simulink model "LogicalAccumulatorModel"  (R2020a)
settings: Solver=FixedStepDiscrete  StartTime=0.0  StopTime=400  FixedStep=0.001  RelTol=1e-3
libraries: AccCellGroup x90
settings Model: Creator=sean  LastModifiedBy=sean
settings OptimizationCC: DefaultParameterBehavior=Inlined  UseDivisionForNetSlopeComputation=on  GainParamInheritBuiltInType=on  UseFloatMulNetSlope=on  InlineInvariantSignals=on  PassReuseOutputArgsAs=Individual arguments  ZeroExternalMemoryAtStartup=off  ZeroInternalMemoryAtStartup=off  NoFixptDivByZeroProtection=on  EfficientFloat2IntCast=on  LifeSpan=1  OptimizeBlockOrder=speed  DifferentSizesBufferReuse=on  EfficientTunableParamExpr=on
settings DebuggingCC: ParameterTunabilityLossMsg=error
settings HardwareCC: ProdBitPerLong=64  ProdLongLongMode=on  ProdHWDeviceType=Intel->x86-64 (Linux 64)
settings SFSimCC: MATLABDynamicMemAlloc=off
settings RTWCC: SystemTargetFile=ert.tlc  GenCodeOnly=on  TemplateMakefile=ert_default_tmf
settings CodeAppCC: ForceParamTrailComments=on  IgnoreCustomStorageClasses=off  OperatorAnnotations=on  SimulinkDataObjDesc=on  SFDataObjDesc=on  CustomSymbolStrGlobalVar=rt$N$M  CustomSymbolStrType=$N$M  CustomSymbolStrFcn=$N$M$F  CustomSymbolStrMacro=$N$M  InsertBlockDesc=on
settings ERTTargetCC: TargetLangStandard=C99 (ISO)  GenerateSampleERTMain=on  IncludeMdlTerminateFcn=off  CombineSignalStateStructs=on  SuppressErrorStatus=on  SupportAbsoluteTime=off  SupportComplex=off  InlinedParameterPlacement=NonHierarchical  ERTCustomFileTemplate=example_file_process.tlc  ERTFilePackagingFormat=CompactWithDataFile

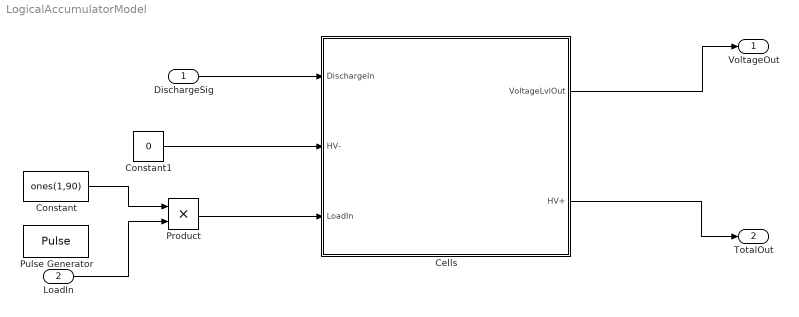
== system LogicalAccumulatorModel ==
  DischargeSig : Inport
  LoadIn : Inport  Port=2
  Cells : Subsystem
  Constant : Constant  Value=ones(1,90)
  Constant1 : Constant  Value=0
  Product : Product
  Pulse Generator : DiscretePulseGenerator  PulseType=Time based  Amplitude=60  Period=300  PulseWidth=99  PhaseDelay=5
  VoltageOut : Outport
  TotalOut : Outport  Port=2
  wires:
  Cells/2(HV+) -> TotalOut/1
  Cells/1(VoltageLvlOut) -> VoltageOut/1
  Constant1/1 -> Cells/2(HV-)
  DischargeSig/1 -> Cells/1(DischargeIn)
  Constant/1 -> Product/1
  Product/1 -> Cells/3(LoadIn)
  LoadIn/1 -> Product/2

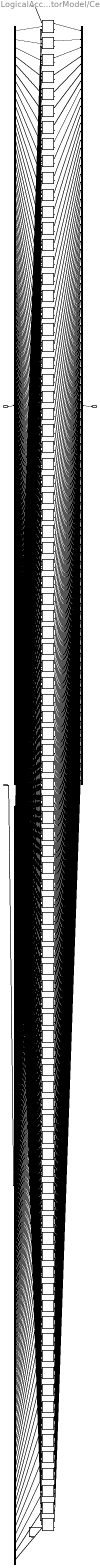
== system LogicalAccumulatorModel/Cells ==
  DischargeIn : Inport
  HV- : Inport  Port=2
  LoadIn : Inport  Port=3
  Cell1 : AccCellGroup/CellGroup  InitialSOCDefficit=0.6400  InternalResistance=0.0018
      settings: SourceProductName=Cell Library
  Cell10 : AccCellGroup/CellGroup  InitialSOCDefficit=0.6500  InternalResistance=0.0018
      settings: SourceProductName=Cell Library
  Cell11 : AccCellGroup/CellGroup  InitialSOCDefficit=0.6100  InternalResistance=0.0018
      settings: SourceProductName=Cell Library
  Cell12 : AccCellGroup/CellGroup  InitialSOCDefficit=0.3900  InternalResistance=0.0018
      settings: SourceProductName=Cell Library
  Cell13 : AccCellGroup/CellGroup  InitialSOCDefficit=0.1400  InternalResistance=0.0018
      settings: SourceProductName=Cell Library
  Cell14 : AccCellGroup/CellGroup  InitialSOCDefficit=0.0200  InternalResistance=0.0018
      settings: SourceProductName=Cell Library
  Cell15 : AccCellGroup/CellGroup  InitialSOCDefficit=0.4200  InternalResistance=0.0018
      settings: SourceProductName=Cell Library
  Cell16 : AccCellGroup/CellGroup  InitialSOCDefficit=0.1800  InternalResistance=0.0018
      settings: SourceProductName=Cell Library
  Cell17 : AccCellGroup/CellGroup  InitialSOCDefficit=0.7300  InternalResistance=0.0018
      settings: SourceProductName=Cell Library
  Cell18 : AccCellGroup/CellGroup  InitialSOCDefficit=0.3700  InternalResistance=0.0018
      settings: SourceProductName=Cell Library
  Cell19 : AccCellGroup/CellGroup  InitialSOCDefficit=0.8400  InternalResistance=0.0018
      settings: SourceProductName=Cell Library
  Cell2 : AccCellGroup/CellGroup  InitialSOCDefficit=0.9600  InternalResistance=0.0018
      settings: SourceProductName=Cell Library
  Cell20 : AccCellGroup/CellGroup  InitialSOCDefficit=0.7400  InternalResistance=0.0018
      settings: SourceProductName=Cell Library
  Cell21 : AccCellGroup/CellGroup  InitialSOCDefficit=0.5700  InternalResistance=0.0018
      settings: SourceProductName=Cell Library
  Cell22 : AccCellGroup/CellGroup  InitialSOCDefficit=0.1700  InternalResistance=0.0018
      settings: SourceProductName=Cell Library
  Cell23 : AccCellGroup/CellGroup  InitialSOCDefficit=0.9600  InternalResistance=0.0018
      settings: SourceProductName=Cell Library
  Cell24 : AccCellGroup/CellGroup  InitialSOCDefficit=0.2600  InternalResistance=0.0018
      settings: SourceProductName=Cell Library
  Cell25 : AccCellGroup/CellGroup  InitialSOCDefficit=0.9300  InternalResistance=0.0018
      settings: SourceProductName=Cell Library
  Cell26 : AccCellGroup/CellGroup  InitialSOCDefficit=0.2200  InternalResistance=0.0018
      settings: SourceProductName=Cell Library
  Cell27 : AccCellGroup/CellGroup  InitialSOCDefficit=0.3700  InternalResistance=0.0018
      settings: SourceProductName=Cell Library
  Cell28 : AccCellGroup/CellGroup  InitialSOCDefficit=0.0800  InternalResistance=0.0018
      settings: SourceProductName=Cell Library
  Cell29 : AccCellGroup/CellGroup  InitialSOCDefficit=0.6400  InternalResistance=0.0018
      settings: SourceProductName=Cell Library
  Cell3 : AccCellGroup/CellGroup  InitialSOCDefficit=0.4400  InternalResistance=0.0018
      settings: SourceProductName=Cell Library
  Cell30 : AccCellGroup/CellGroup  InitialSOCDefficit=0.1800  InternalResistance=0.0018
      settings: SourceProductName=Cell Library
  Cell31 : AccCellGroup/CellGroup  InitialSOCDefficit=0.0400  InternalResistance=0.0018
      settings: SourceProductName=Cell Library
  Cell32 : AccCellGroup/CellGroup  InitialSOCDefficit=0.7300  InternalResistance=0.0018
      settings: SourceProductName=Cell Library
  Cell33 : AccCellGroup/CellGroup  InitialSOCDefficit=0.3500  InternalResistance=0.0018
      settings: SourceProductName=Cell Library
  Cell34 : AccCellGroup/CellGroup  InitialSOCDefficit=0.6600  InternalResistance=0.0018
      settings: SourceProductName=Cell Library
  Cell35 : AccCellGroup/CellGroup  InitialSOCDefficit=0.3800  InternalResistance=0.0018
      settings: SourceProductName=Cell Library
  Cell36 : AccCellGroup/CellGroup  InitialSOCDefficit=0.6300  InternalResistance=0.0018
      settings: SourceProductName=Cell Library
  Cell37 : AccCellGroup/CellGroup  InitialSOCDefficit=0.0200  InternalResistance=0.0018
      settings: SourceProductName=Cell Library
  Cell38 : AccCellGroup/CellGroup  InitialSOCDefficit=0.9100  InternalResistance=0.0018
      settings: SourceProductName=Cell Library
  Cell39 : AccCellGroup/CellGroup  InitialSOCDefficit=0.8000  InternalResistance=0.0018
      settings: SourceProductName=Cell Library
  Cell4 : AccCellGroup/CellGroup  InitialSOCDefficit=0.0600  InternalResistance=0.0018
      settings: SourceProductName=Cell Library
  Cell40 : AccCellGroup/CellGroup  InitialSOCDefficit=0.7500  InternalResistance=0.0018
      settings: SourceProductName=Cell Library
  Cell41 : AccCellGroup/CellGroup  InitialSOCDefficit=0.8200  InternalResistance=0.0018
      settings: SourceProductName=Cell Library
  Cell42 : AccCellGroup/CellGroup  InitialSOCDefficit=0.3800  InternalResistance=0.0018
      settings: SourceProductName=Cell Library
  Cell43 : AccCellGroup/CellGroup  InitialSOCDefficit=0.6200  InternalResistance=0.0018
      settings: SourceProductName=Cell Library
  Cell44 : AccCellGroup/CellGroup  InitialSOCDefficit=0.5800  InternalResistance=0.0018
      settings: SourceProductName=Cell Library
  Cell45 : AccCellGroup/CellGroup  InitialSOCDefficit=0.5300  InternalResistance=0.0018
      settings: SourceProductName=Cell Library
  Cell46 : AccCellGroup/CellGroup  InitialSOCDefficit=0.2700  InternalResistance=0.0018
      settings: SourceProductName=Cell Library
  Cell47 : AccCellGroup/CellGroup  InitialSOCDefficit=0.2500  InternalResistance=0.0018
      settings: SourceProductName=Cell Library
  Cell48 : AccCellGroup/CellGroup  InitialSOCDefficit=0.4500  InternalResistance=0.0018
      settings: SourceProductName=Cell Library
  Cell49 : AccCellGroup/CellGroup  InitialSOCDefficit=0.2200  InternalResistance=0.0018
      settings: SourceProductName=Cell Library
  Cell5 : AccCellGroup/CellGroup  InitialSOCDefficit=0.8700  InternalResistance=0.0018
      settings: SourceProductName=Cell Library
  Cell50 : AccCellGroup/CellGroup  InitialSOCDefficit=0.8100  InternalResistance=0.0018
      settings: SourceProductName=Cell Library
  Cell{51,56,75,78} (4 alike) : AccCellGroup/CellGroup  InitialSOCDefficit=0.9900  InternalResistance=0.0018
      settings: SourceProductName=Cell Library
  Cell52 : AccCellGroup/CellGroup  InitialSOCDefficit=0.0300  InternalResistance=0.0018
      settings: SourceProductName=Cell Library
  Cell53 : AccCellGroup/CellGroup  InitialSOCDefficit=0.5400  InternalResistance=0.0018
      settings: SourceProductName=Cell Library
  Cell54 : AccCellGroup/CellGroup  InitialSOCDefficit=0.0800  InternalResistance=0.0018
      settings: SourceProductName=Cell Library
  Cell55 : AccCellGroup/CellGroup  InitialSOCDefficit=0.8100  InternalResistance=0.0018
      settings: SourceProductName=Cell Library
  Cell57 : AccCellGroup/CellGroup  InitialSOCDefficit=0.0600  InternalResistance=0.0018
      settings: SourceProductName=Cell Library
  Cell58 : AccCellGroup/CellGroup  InitialSOCDefficit=0.9400  InternalResistance=0.0018
      settings: SourceProductName=Cell Library
  Cell59 : AccCellGroup/CellGroup  InitialSOCDefficit=0.0100  InternalResistance=0.0018
      settings: SourceProductName=Cell Library
  Cell6 : AccCellGroup/CellGroup  InitialSOCDefficit=0.6300  InternalResistance=0.0018
      settings: SourceProductName=Cell Library
  Cell60 : AccCellGroup/CellGroup  InitialSOCDefficit=0.6900  InternalResistance=0.0018
      settings: SourceProductName=Cell Library
  Cell61 : AccCellGroup/CellGroup  InitialSOCDefficit=0.7900  InternalResistance=0.0018
      settings: SourceProductName=Cell Library
  Cell62 : AccCellGroup/CellGroup  InitialSOCDefficit=0.5300  InternalResistance=0.0018
      settings: SourceProductName=Cell Library
  Cell63 : AccCellGroup/CellGroup  InitialSOCDefficit=0.8900  InternalResistance=0.0018
      settings: SourceProductName=Cell Library
  Cell64 : AccCellGroup/CellGroup  InitialSOCDefficit=0.9000  InternalResistance=0.0018
      settings: SourceProductName=Cell Library
  Cell65 : AccCellGroup/CellGroup  InitialSOCDefficit=0.6300  InternalResistance=0.0018
      settings: SourceProductName=Cell Library
  Cell66 : AccCellGroup/CellGroup  InitialSOCDefficit=0.1300  InternalResistance=0.0018
      settings: SourceProductName=Cell Library
  Cell67 : AccCellGroup/CellGroup  InitialSOCDefficit=0.2100  InternalResistance=0.0018
      settings: SourceProductName=Cell Library
  Cell68 : AccCellGroup/CellGroup  InitialSOCDefficit=0.1800  InternalResistance=0.0018
      settings: SourceProductName=Cell Library
  Cell69 : AccCellGroup/CellGroup  InitialSOCDefficit=0.0400  InternalResistance=0.0018
      settings: SourceProductName=Cell Library
  Cell7 : AccCellGroup/CellGroup  InitialSOCDefficit=0.3500  InternalResistance=0.0018
      settings: SourceProductName=Cell Library
  Cell70 : AccCellGroup/CellGroup  InitialSOCDefficit=0.1000  InternalResistance=0.0018
      settings: SourceProductName=Cell Library
  Cell71 : AccCellGroup/CellGroup  InitialSOCDefficit=0.6200  InternalResistance=0.0018
      settings: SourceProductName=Cell Library
  Cell72 : AccCellGroup/CellGroup  InitialSOCDefficit=0.9400  InternalResistance=0.0018
      settings: SourceProductName=Cell Library
  Cell73 : AccCellGroup/CellGroup  InitialSOCDefficit=0.3500  InternalResistance=0.0018
      settings: SourceProductName=Cell Library
  Cell74 : AccCellGroup/CellGroup  InitialSOCDefficit=0.4100  InternalResistance=0.0018
      settings: SourceProductName=Cell Library
  Cell76 : AccCellGroup/CellGroup  InitialSOCDefficit=0.9500  InternalResistance=0.0018
      settings: SourceProductName=Cell Library
  Cell77 : AccCellGroup/CellGroup  InitialSOCDefficit=0.6800  InternalResistance=0.0018
      settings: SourceProductName=Cell Library
  Cell79 : AccCellGroup/CellGroup  InitialSOCDefficit=0.7700  InternalResistance=0.0018
      settings: SourceProductName=Cell Library
  Cell8 : AccCellGroup/CellGroup  InitialSOCDefficit=1.0000  InternalResistance=0.0018
      settings: SourceProductName=Cell Library
  Cell80 : AccCellGroup/CellGroup  InitialSOCDefficit=0.3400  InternalResistance=0.0018
      settings: SourceProductName=Cell Library
  Cell81 : AccCellGroup/CellGroup  InitialSOCDefficit=0.6600  InternalResistance=0.0018
      settings: SourceProductName=Cell Library
  Cell82 : AccCellGroup/CellGroup  InitialSOCDefficit=0.2400  InternalResistance=0.0018
      settings: SourceProductName=Cell Library
  Cell83 : AccCellGroup/CellGroup  InitialSOCDefficit=0.2900  InternalResistance=0.0018
      settings: SourceProductName=Cell Library
  Cell84 : AccCellGroup/CellGroup  InitialSOCDefficit=0.6800  InternalResistance=0.0018
      settings: SourceProductName=Cell Library
  Cell85 : AccCellGroup/CellGroup  InitialSOCDefficit=0.5300  InternalResistance=0.0018
      settings: SourceProductName=Cell Library
  Cell86 : AccCellGroup/CellGroup  InitialSOCDefficit=0.4100  InternalResistance=0.0018
      settings: SourceProductName=Cell Library
  Cell87 : AccCellGroup/CellGroup  InitialSOCDefficit=0.6000  InternalResistance=0.0018
      settings: SourceProductName=Cell Library
  Cell88 : AccCellGroup/CellGroup  InitialSOCDefficit=0.7500  InternalResistance=0.0018
      settings: SourceProductName=Cell Library
  Cell89 : AccCellGroup/CellGroup  InitialSOCDefficit=0.5800  InternalResistance=0.0018
      settings: SourceProductName=Cell Library
  Cell9 : AccCellGroup/CellGroup  InitialSOCDefficit=0.2200  InternalResistance=0.0018
      settings: SourceProductName=Cell Library
  Cell90 : AccCellGroup/CellGroup  InitialSOCDefficit=0.5500  InternalResistance=0.0018
      settings: SourceProductName=Cell Library
  DischargeMux : Demux  Outputs=90
  LoadMux : Demux  Outputs=90
  VoltageMux : Mux  Inputs=90
  VoltageLvlOut : Outport
  HV+ : Outport  Port=2
  wires:
  DischargeMux/1 -> Cell1/2
  Cell1/1 -> VoltageMux/1
  LoadMux/1 -> Cell1/3
  DischargeMux/2 -> Cell2/2
  Cell2/1 -> VoltageMux/2
  LoadMux/2 -> Cell2/3
  Cell1/2 -> Cell2/1
  DischargeMux/3 -> Cell3/2
  Cell3/1 -> VoltageMux/3
  LoadMux/3 -> Cell3/3
  Cell2/2 -> Cell3/1
  DischargeMux/4 -> Cell4/2
  Cell4/1 -> VoltageMux/4
  LoadMux/4 -> Cell4/3
  Cell3/2 -> Cell4/1
  DischargeMux/5 -> Cell5/2
  Cell5/1 -> VoltageMux/5
  LoadMux/5 -> Cell5/3
  Cell4/2 -> Cell5/1
  DischargeMux/6 -> Cell6/2
  Cell6/1 -> VoltageMux/6
  LoadMux/6 -> Cell6/3
  Cell5/2 -> Cell6/1
  DischargeMux/7 -> Cell7/2
  Cell7/1 -> VoltageMux/7
  LoadMux/7 -> Cell7/3
  Cell6/2 -> Cell7/1
  DischargeMux/8 -> Cell8/2
  Cell8/1 -> VoltageMux/8
  LoadMux/8 -> Cell8/3
  Cell7/2 -> Cell8/1
  DischargeMux/9 -> Cell9/2
  Cell9/1 -> VoltageMux/9
  LoadMux/9 -> Cell9/3
  Cell8/2 -> Cell9/1
  DischargeMux/10 -> Cell10/2
  Cell10/1 -> VoltageMux/10
  LoadMux/10 -> Cell10/3
  Cell9/2 -> Cell10/1
  DischargeMux/11 -> Cell11/2
  Cell11/1 -> VoltageMux/11
  LoadMux/11 -> Cell11/3
  Cell10/2 -> Cell11/1
  DischargeMux/12 -> Cell12/2
  Cell12/1 -> VoltageMux/12
  LoadMux/12 -> Cell12/3
  Cell11/2 -> Cell12/1
  DischargeMux/13 -> Cell13/2
  Cell13/1 -> VoltageMux/13
  LoadMux/13 -> Cell13/3
  Cell12/2 -> Cell13/1
  DischargeMux/14 -> Cell14/2
  Cell14/1 -> VoltageMux/14
  LoadMux/14 -> Cell14/3
  Cell13/2 -> Cell14/1
  DischargeMux/15 -> Cell15/2
  Cell15/1 -> VoltageMux/15
  LoadMux/15 -> Cell15/3
  Cell14/2 -> Cell15/1
  DischargeMux/16 -> Cell16/2
  Cell16/1 -> VoltageMux/16
  LoadMux/16 -> Cell16/3
  Cell15/2 -> Cell16/1
  DischargeMux/17 -> Cell17/2
  Cell17/1 -> VoltageMux/17
  LoadMux/17 -> Cell17/3
  Cell16/2 -> Cell17/1
  DischargeMux/18 -> Cell18/2
  Cell18/1 -> VoltageMux/18
  LoadMux/18 -> Cell18/3
  Cell17/2 -> Cell18/1
  DischargeMux/19 -> Cell19/2
  Cell19/1 -> VoltageMux/19
  LoadMux/19 -> Cell19/3
  Cell18/2 -> Cell19/1
  DischargeMux/20 -> Cell20/2
  Cell20/1 -> VoltageMux/20
  LoadMux/20 -> Cell20/3
  Cell19/2 -> Cell20/1
  DischargeMux/21 -> Cell21/2
  Cell21/1 -> VoltageMux/21
  LoadMux/21 -> Cell21/3
  Cell20/2 -> Cell21/1
  DischargeMux/22 -> Cell22/2
  Cell22/1 -> VoltageMux/22
  LoadMux/22 -> Cell22/3
  Cell21/2 -> Cell22/1
  DischargeMux/23 -> Cell23/2
  Cell23/1 -> VoltageMux/23
  LoadMux/23 -> Cell23/3
  Cell22/2 -> Cell23/1
  DischargeMux/24 -> Cell24/2
  Cell24/1 -> VoltageMux/24
  LoadMux/24 -> Cell24/3
  Cell23/2 -> Cell24/1
  DischargeMux/25 -> Cell25/2
  Cell25/1 -> VoltageMux/25
  LoadMux/25 -> Cell25/3
  Cell24/2 -> Cell25/1
  DischargeMux/26 -> Cell26/2
  Cell26/1 -> VoltageMux/26
  LoadMux/26 -> Cell26/3
  Cell25/2 -> Cell26/1
  DischargeMux/27 -> Cell27/2
  Cell27/1 -> VoltageMux/27
  LoadMux/27 -> Cell27/3
  Cell26/2 -> Cell27/1
  DischargeMux/28 -> Cell28/2
  Cell28/1 -> VoltageMux/28
  LoadMux/28 -> Cell28/3
  Cell27/2 -> Cell28/1
  DischargeMux/29 -> Cell29/2
  Cell29/1 -> VoltageMux/29
  LoadMux/29 -> Cell29/3
  Cell28/2 -> Cell29/1
  DischargeMux/30 -> Cell30/2
  Cell30/1 -> VoltageMux/30
  LoadMux/30 -> Cell30/3
  Cell29/2 -> Cell30/1
  DischargeMux/31 -> Cell31/2
  Cell31/1 -> VoltageMux/31
  LoadMux/31 -> Cell31/3
  Cell30/2 -> Cell31/1
  DischargeMux/32 -> Cell32/2
  Cell32/1 -> VoltageMux/32
  LoadMux/32 -> Cell32/3
  Cell31/2 -> Cell32/1
  DischargeMux/33 -> Cell33/2
  Cell33/1 -> VoltageMux/33
  LoadMux/33 -> Cell33/3
  Cell32/2 -> Cell33/1
  DischargeMux/34 -> Cell34/2
  Cell34/1 -> VoltageMux/34
  LoadMux/34 -> Cell34/3
  Cell33/2 -> Cell34/1
  DischargeMux/35 -> Cell35/2
  Cell35/1 -> VoltageMux/35
  LoadMux/35 -> Cell35/3
  Cell34/2 -> Cell35/1
  DischargeMux/36 -> Cell36/2
  Cell36/1 -> VoltageMux/36
  LoadMux/36 -> Cell36/3
  Cell35/2 -> Cell36/1
  DischargeMux/37 -> Cell37/2
  Cell37/1 -> VoltageMux/37
  LoadMux/37 -> Cell37/3
  Cell36/2 -> Cell37/1
  DischargeMux/38 -> Cell38/2
  Cell38/1 -> VoltageMux/38
  LoadMux/38 -> Cell38/3
  Cell37/2 -> Cell38/1
  DischargeMux/39 -> Cell39/2
  Cell39/1 -> VoltageMux/39
  LoadMux/39 -> Cell39/3
  Cell38/2 -> Cell39/1
  DischargeMux/40 -> Cell40/2
  Cell40/1 -> VoltageMux/40
  LoadMux/40 -> Cell40/3
  Cell39/2 -> Cell40/1
  DischargeMux/41 -> Cell41/2
  Cell41/1 -> VoltageMux/41
  LoadMux/41 -> Cell41/3
  Cell40/2 -> Cell41/1
  DischargeMux/42 -> Cell42/2
  Cell42/1 -> VoltageMux/42
  LoadMux/42 -> Cell42/3
  Cell41/2 -> Cell42/1
  DischargeMux/43 -> Cell43/2
  Cell43/1 -> VoltageMux/43
  LoadMux/43 -> Cell43/3
  Cell42/2 -> Cell43/1
  DischargeMux/44 -> Cell44/2
  Cell44/1 -> VoltageMux/44
  LoadMux/44 -> Cell44/3
  Cell43/2 -> Cell44/1
  DischargeMux/45 -> Cell45/2
  Cell45/1 -> VoltageMux/45
  LoadMux/45 -> Cell45/3
  Cell44/2 -> Cell45/1
  DischargeMux/46 -> Cell46/2
  Cell46/1 -> VoltageMux/46
  LoadMux/46 -> Cell46/3
  Cell45/2 -> Cell46/1
  DischargeMux/47 -> Cell47/2
  Cell47/1 -> VoltageMux/47
  LoadMux/47 -> Cell47/3
  Cell46/2 -> Cell47/1
  DischargeMux/48 -> Cell48/2
  Cell48/1 -> VoltageMux/48
  LoadMux/48 -> Cell48/3
  Cell47/2 -> Cell48/1
  DischargeMux/49 -> Cell49/2
  Cell49/1 -> VoltageMux/49
  LoadMux/49 -> Cell49/3
  Cell48/2 -> Cell49/1
  DischargeMux/50 -> Cell50/2
  Cell50/1 -> VoltageMux/50
  LoadMux/50 -> Cell50/3
  Cell49/2 -> Cell50/1
  DischargeMux/51 -> Cell51/2
  Cell51/1 -> VoltageMux/51
  LoadMux/51 -> Cell51/3
  Cell50/2 -> Cell51/1
  DischargeMux/52 -> Cell52/2
  Cell52/1 -> VoltageMux/52
  LoadMux/52 -> Cell52/3
  Cell51/2 -> Cell52/1
  DischargeMux/53 -> Cell53/2
  Cell53/1 -> VoltageMux/53
  LoadMux/53 -> Cell53/3
  Cell52/2 -> Cell53/1
  DischargeMux/54 -> Cell54/2
  Cell54/1 -> VoltageMux/54
  LoadMux/54 -> Cell54/3
  Cell53/2 -> Cell54/1
  DischargeMux/55 -> Cell55/2
  Cell55/1 -> VoltageMux/55
  LoadMux/55 -> Cell55/3
  Cell54/2 -> Cell55/1
  DischargeMux/56 -> Cell56/2
  Cell56/1 -> VoltageMux/56
  LoadMux/56 -> Cell56/3
  Cell55/2 -> Cell56/1
  DischargeMux/57 -> Cell57/2
  Cell57/1 -> VoltageMux/57
  LoadMux/57 -> Cell57/3
  Cell56/2 -> Cell57/1
  DischargeMux/58 -> Cell58/2
  Cell58/1 -> VoltageMux/58
  LoadMux/58 -> Cell58/3
  Cell57/2 -> Cell58/1
  DischargeMux/59 -> Cell59/2
  Cell59/1 -> VoltageMux/59
  LoadMux/59 -> Cell59/3
  Cell58/2 -> Cell59/1
  DischargeMux/60 -> Cell60/2
  Cell60/1 -> VoltageMux/60
  LoadMux/60 -> Cell60/3
  Cell59/2 -> Cell60/1
  DischargeMux/61 -> Cell61/2
  Cell61/1 -> VoltageMux/61
  LoadMux/61 -> Cell61/3
  Cell60/2 -> Cell61/1
  DischargeMux/62 -> Cell62/2
  Cell62/1 -> VoltageMux/62
  LoadMux/62 -> Cell62/3
  Cell61/2 -> Cell62/1
  DischargeMux/63 -> Cell63/2
  Cell63/1 -> VoltageMux/63
  LoadMux/63 -> Cell63/3
  Cell62/2 -> Cell63/1
  DischargeMux/64 -> Cell64/2
  Cell64/1 -> VoltageMux/64
  LoadMux/64 -> Cell64/3
  Cell63/2 -> Cell64/1
  DischargeMux/65 -> Cell65/2
  Cell65/1 -> VoltageMux/65
  LoadMux/65 -> Cell65/3
  Cell64/2 -> Cell65/1
  DischargeMux/66 -> Cell66/2
  Cell66/1 -> VoltageMux/66
  LoadMux/66 -> Cell66/3
  Cell65/2 -> Cell66/1
  DischargeMux/67 -> Cell67/2
  Cell67/1 -> VoltageMux/67
  LoadMux/67 -> Cell67/3
  Cell66/2 -> Cell67/1
  DischargeMux/68 -> Cell68/2
  Cell68/1 -> VoltageMux/68
  LoadMux/68 -> Cell68/3
  Cell67/2 -> Cell68/1
  DischargeMux/69 -> Cell69/2
  Cell69/1 -> VoltageMux/69
  LoadMux/69 -> Cell69/3
  Cell68/2 -> Cell69/1
  DischargeMux/70 -> Cell70/2
  Cell70/1 -> VoltageMux/70
  LoadMux/70 -> Cell70/3
  Cell69/2 -> Cell70/1
  DischargeMux/71 -> Cell71/2
  Cell71/1 -> VoltageMux/71
  LoadMux/71 -> Cell71/3
  Cell70/2 -> Cell71/1
  DischargeMux/72 -> Cell72/2
  Cell72/1 -> VoltageMux/72
  LoadMux/72 -> Cell72/3
  Cell71/2 -> Cell72/1
  DischargeMux/73 -> Cell73/2
  Cell73/1 -> VoltageMux/73
  LoadMux/73 -> Cell73/3
  Cell72/2 -> Cell73/1
  DischargeMux/74 -> Cell74/2
  Cell74/1 -> VoltageMux/74
  LoadMux/74 -> Cell74/3
  Cell73/2 -> Cell74/1
  DischargeMux/75 -> Cell75/2
  Cell75/1 -> VoltageMux/75
  LoadMux/75 -> Cell75/3
  Cell74/2 -> Cell75/1
  DischargeMux/76 -> Cell76/2
  Cell76/1 -> VoltageMux/76
  LoadMux/76 -> Cell76/3
  Cell75/2 -> Cell76/1
  DischargeMux/77 -> Cell77/2
  Cell77/1 -> VoltageMux/77
  LoadMux/77 -> Cell77/3
  Cell76/2 -> Cell77/1
  DischargeMux/78 -> Cell78/2
  Cell78/1 -> VoltageMux/78
  LoadMux/78 -> Cell78/3
  Cell77/2 -> Cell78/1
  DischargeMux/79 -> Cell79/2
  Cell79/1 -> VoltageMux/79
  LoadMux/79 -> Cell79/3
  Cell78/2 -> Cell79/1
  DischargeMux/80 -> Cell80/2
  Cell80/1 -> VoltageMux/80
  LoadMux/80 -> Cell80/3
  Cell79/2 -> Cell80/1
  DischargeMux/81 -> Cell81/2
  Cell81/1 -> VoltageMux/81
  LoadMux/81 -> Cell81/3
  Cell80/2 -> Cell81/1
  DischargeMux/82 -> Cell82/2
  Cell82/1 -> VoltageMux/82
  LoadMux/82 -> Cell82/3
  Cell81/2 -> Cell82/1
  DischargeMux/83 -> Cell83/2
  Cell83/1 -> VoltageMux/83
  LoadMux/83 -> Cell83/3
  Cell82/2 -> Cell83/1
  DischargeMux/84 -> Cell84/2
  Cell84/1 -> VoltageMux/84
  LoadMux/84 -> Cell84/3
  Cell83/2 -> Cell84/1
  DischargeMux/85 -> Cell85/2
  Cell85/1 -> VoltageMux/85
  LoadMux/85 -> Cell85/3
  Cell84/2 -> Cell85/1
  DischargeMux/86 -> Cell86/2
  Cell86/1 -> VoltageMux/86
  LoadMux/86 -> Cell86/3
  Cell85/2 -> Cell86/1
  DischargeMux/87 -> Cell87/2
  Cell87/1 -> VoltageMux/87
  LoadMux/87 -> Cell87/3
  Cell86/2 -> Cell87/1
  DischargeMux/88 -> Cell88/2
  Cell88/1 -> VoltageMux/88
  LoadMux/88 -> Cell88/3
  Cell87/2 -> Cell88/1
  DischargeMux/89 -> Cell89/2
  Cell89/1 -> VoltageMux/89
  LoadMux/89 -> Cell89/3
  Cell88/2 -> Cell89/1
  DischargeMux/90 -> Cell90/2
  Cell90/1 -> VoltageMux/90
  LoadMux/90 -> Cell90/3
  Cell89/2 -> Cell90/1
  HV-/1 -> Cell1/1
  Cell90/2 -> HV+/1
  LoadIn/1 -> LoadMux/1
  DischargeIn/1 -> DischargeMux/1
  VoltageMux/1 -> VoltageLvlOut/1
